simulink model "simulation"  (R2023b)
settings: Solver=ode45  StartTime=0.0  StopTime=0.2  MaxStep=1.176e-08  RelTol=1e-3  EnableMultiTasking=on
libraries: spsSeriesRLCBranchLib x5, spsDiodeLib x4, spsMosfetLib x4, spsCurrentMeasurementLib x3, spsVoltageMeasurementLib x3, spsDCVoltageSourceLib x1, spsMutualInductanceLib x1, spspowerguiLib x1
settings Model: Creator=hitwyz  LastModifiedBy=Lenovo
settings SolverCC: AlgebraicLoopSolver=TrustRegion
settings DataIOCC: LimitDataPoints=on  SaveFormat=Array  ReturnWorkspaceOutputs=off
settings OptimizationCC: LifeSpan=inf
settings DebuggingCC: SolverPrmCheckMsg=warning  UnconnectedInputMsg=warning  UnconnectedOutputMsg=warning  UnconnectedLineMsg=warning  SFUnexpectedBacktrackingDiag=warning  SFNoUnconditionalDefaultTransitionDiag=warning  SFExecutionAtInitializationDiag=none  ArithmeticOperatorsInVariantConditions=warning
settings HardwareCC: ProdBitPerPointer=32  ProdBitPerSizeT=32  ProdBitPerPtrDiffT=32  ProdLargestAtomicFloat=None  ProdIntDivRoundTo=Undefined  ProdEndianess=Unspecified  ProdWordSize=32  ProdHWDeviceType=32-bit Generic
settings ModelReferenceCC: EnableRefExpFcnMdlSchedulingChecks=on  PropagateSignalLabelsOutOfModel=off
settings SFSimCC: SimUseLocalCustomCode=off  CustomCodeUndefinedFunction=UseInterfaceOnly
settings RTWCC: RTWUseLocalCustomCode=off  DLArmComputeVersion=19.05
settings CodeAppCC: StateflowObjectComments=on
settings GRTTargetCC: TargetLangStandard=C89/C90 (ANSI)
settings ConfigComp: CovMetricSettings=dw  CovSaveCumulativeToWorkspaceVar=on  CovSaveSingleToWorkspaceVar=on  CovExternalEMLEnable=off  CovSFcnEnable=off
settings SimscapeCC: SimscapeNormalizeSystem=off

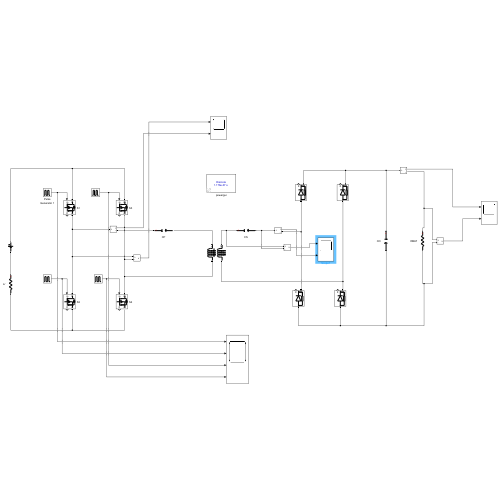
[thumbnail: Simulink's stored preview of the top-level diagram]
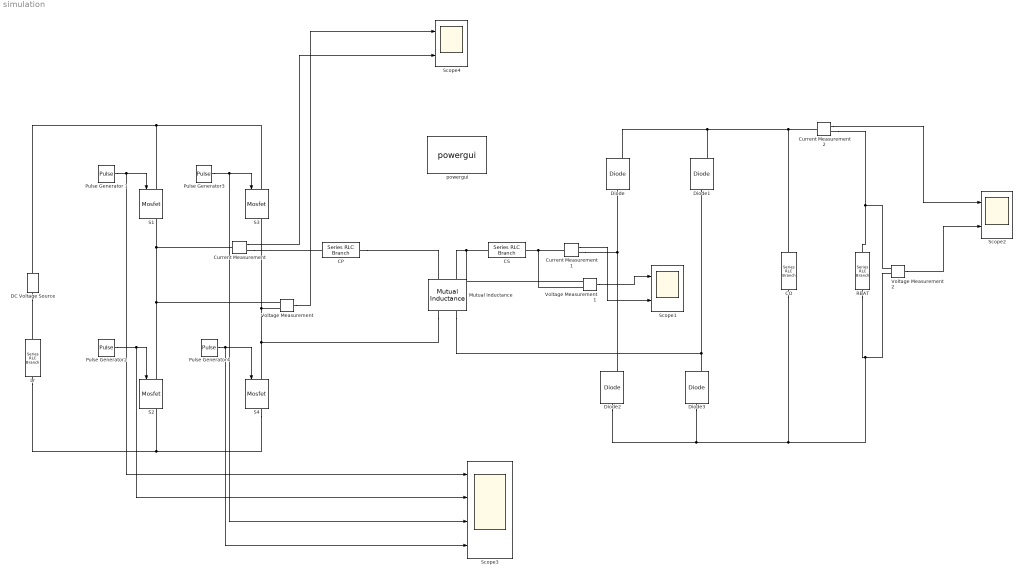
== system simulation ==
  CO : spsSeriesRLCBranchLib/Series RLC Branch  LConnTagsString=__new0  RConnTagsString=__new0  BranchType=C  Resistance=1  Inductance=1e-3  SetiL0=off  InitialCurrent=0  Capacitance=1000e-6  Setx0=off  InitialVoltage=0  Measurements=None
  CP : spsSeriesRLCBranchLib/Series RLC Branch  LConnTagsString=__new0  RConnTagsString=__new0  BranchType=C  Resistance=1  Inductance=1e-3  SetiL0=off  InitialCurrent=0  Capacitance=287.3e-9  Setx0=on  InitialVoltage=0  Measurements=None
  CS : spsSeriesRLCBranchLib/Series RLC Branch  LConnTagsString=__new0  RConnTagsString=__new0  BranchType=C  Resistance=1  Inductance=1e-3  SetiL0=off  InitialCurrent=0  Capacitance=287.3e-9  Setx0=off  InitialVoltage=0  Measurements=None
  Current Measurement : spsCurrentMeasurementLib/Current Measurement  PhasorSimulation=off  OutputType=Complex  PSBequivalent=0
  Current Measurement1 : spsCurrentMeasurementLib/Current Measurement  PhasorSimulation=off  OutputType=Complex  PSBequivalent=0
  Current Measurement2 : spsCurrentMeasurementLib/Current Measurement  PhasorSimulation=off  OutputType=Complex  PSBequivalent=0
  DC Voltage Source : spsDCVoltageSourceLib/DC Voltage Source  Amplitude=125  Measurements=None
  Diode{,1..3} (4 alike) : spsDiodeLib/Diode  Ron=0.001  Lon=0  Vf=0.8  IC=0  UseSnubber=0  Rs=500  Cs=250e-9  Measurements=on
  Lr : spsSeriesRLCBranchLib/Series RLC Branch  LConnTagsString=__new0  RConnTagsString=__new0  BranchType=R  Resistance=1e-05  Inductance=1e-3  SetiL0=off  InitialCurrent=0  Capacitance=37.3e-9  Setx0=off  InitialVoltage=0  Measurements=None
  Mutual Inductance : spsMutualInductanceLib/Mutual Inductance  LConnTagsString=a|b  RConnTagsString=A|B  TypeOfMutual=Two or three windings with equal mutual terms  NumberOfWindings=3  SelfImpedance1=[0 61.207710e-06]  SelfImpedance2=[0 61.375513e-06]  ThreeWindings=off  SelfImpedance3=[ 1.1 1.1e-03]  MutualImpedance=[0 46.061839e-06]  InductanceMatrix="[1.0 0.9  0.9 ;  0.9 1.0  0.9;  0.9 0.9 1.0 ] * 1e-3"  ResistanceMatrix="[1.0 0.9  0.9 ;  0.9 1.0  0.9;  0.9 0.9 1.0 ]"  Measurements=None
  Pulse Generator 1 : DiscretePulseGenerator  PulseType=Time based  Period=1/85000  PulseWidth=50
  Pulse Generator2 : DiscretePulseGenerator  PulseType=Time based  Period=1/85000  PulseWidth=50  PhaseDelay=0.5/85000
  Pulse Generator3 : DiscretePulseGenerator  PulseType=Time based  Period=1/85000  PulseWidth=50  PhaseDelay=0.5/85000
  Pulse Generator4 : DiscretePulseGenerator  PulseType=Time based  Period=1/85000  PulseWidth=50
  RBAT : spsSeriesRLCBranchLib/Series RLC Branch  LConnTagsString=__new0  RConnTagsString=__new0  BranchType=R  Resistance=33.33  Inductance=1e-3  SetiL0=off  InitialCurrent=0  Capacitance=37.3e-9  Setx0=off  InitialVoltage=0  Measurements=None
  S{1..4} (4 alike) : spsMosfetLib/Mosfet  Ron=0.1  Lon=0  Rd=0.01  Vfd=0  IC=0  Rs=1e5  Cs=inf  Measurements=on
  Scope1 : Scope  NumInputPorts=2
  Scope2 : Scope  NumInputPorts=2
  Scope3 : Scope  NumInputPorts=4
  Scope4 : Scope  NumInputPorts=2
  Voltage Measurement : spsVoltageMeasurementLib/Voltage Measurement  PhasorSimulation=off  OutputType=Complex  PSBequivalent=0
  Voltage Measurement1 : spsVoltageMeasurementLib/Voltage Measurement  PhasorSimulation=off  OutputType=Complex  PSBequivalent=0
  Voltage Measurement2 : spsVoltageMeasurementLib/Voltage Measurement  PhasorSimulation=off  OutputType=Complex  PSBequivalent=0
  powergui : spspowerguiLib/powergui  Priority=1  SimulationMode=Discrete  SampleTime=1/85000/100  frequency=60  Iterations=50  frequencyindice=0  Pbase=100e6  ErrMax=1e-4  UnitsV=kV  UnitsW=MW  buscounter=0  FunctionMessages=off  echomessages=off  EnableUseOfTLC=off  CurrentSourceSwitches=off  DisableSnubberDevices=off  DisableRonSwitches=off  DisableVfSwitches=off  DisplayEquations=off  AutomaticDiscreteSolvers=off  SolverType=Tustin  Interpol=off  ExternalGateDelay=off  methode=off  Ts=0  x0status=blocks  SPID=off  SwTol=0  HookPort=off  NonlinearTolerance=1e-4  nMaxIteration=100  ContinueOnMaxIteration=off  RestoreLinks=warning  ResistiveCurrentMeasurement=off  Frange=[0:2:500]  Ylog=off  Xlog=on  ShowGrid=off  save=off  variable=ZData  structure=0  ZoomFFT=off  StartTime=0.0  cycles=1  DisplayStyle=1  fundamental=60  FreqAxis=off  MaxFrequency=1000  frequencyindicesteady=1  RmsSteady=1  display=off
  wires:
  Pulse Generator 1/1 -> Scope3/1, S1/1
  Pulse Generator3/1 -> Scope3/3, S3/1
  Pulse Generator2/1 -> Scope3/2, S2/1
  Pulse Generator4/1 -> Scope3/4, S4/1
  Voltage Measurement/1 -> Scope4/1
  Current Measurement/1 -> Scope4/2
  Voltage Measurement1/1 -> Scope1/1
  Current Measurement1/1 -> Scope1/2
  Current Measurement2/1 -> Scope2/1
  Voltage Measurement2/1 -> Scope2/2
  connections:
  S2/LConn1 -- Current Measurement/LConn1 -- S1/RConn1 -- Voltage Measurement/LConn1
  S4/LConn1 -- Mutual Inductance/RConn1 -- Voltage Measurement/LConn2 -- S3/RConn1
  DC Voltage Source/RConn1 -- S1/LConn1 -- S3/LConn1
  S4/RConn1 -- Lr/RConn1 -- S2/RConn1
  CP/RConn1 -- Mutual Inductance/LConn1
  Mutual Inductance/LConn2 -- Voltage Measurement1/LConn1 -- CS/LConn1
  CO/LConn1 -- Diode1/RConn1 -- Diode/RConn1 -- Current Measurement2/LConn1
  Voltage Measurement2/LConn2 -- Diode2/LConn1 -- Diode3/LConn1 -- CO/RConn1 -- RBAT/RConn1
  Current Measurement/RConn1 -- CP/LConn1
  Current Measurement2/RConn1 -- RBAT/LConn1 -- Voltage Measurement2/LConn1
  DC Voltage Source/LConn1 -- Lr/LConn1
  Diode2/RConn1 -- Current Measurement1/RConn1 -- Diode/LConn1
  Diode3/RConn1 -- Mutual Inductance/RConn2 -- Diode1/LConn1
  Current Measurement1/LConn1 -- Voltage Measurement1/LConn2 -- CS/RConn1
